simulink library "SignalPreprocessingLib"  (R2020b)
settings: Solver=VariableStepAuto  StartTime=0.0  StopTime=10.0  RelTol=1e-3
undefined symbols (not defined in the file or in its folder): fdesignblkfcn, fs, gcbh, param_ecg_gain_mv
(part 1 of 7)
settings Model: Creator=Rafael  LastModifiedBy=Rafael

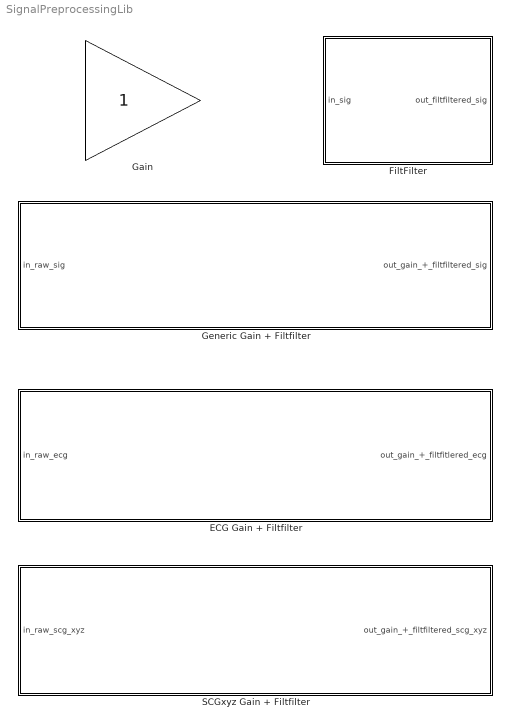
== system SignalPreprocessingLib ==
  ECG Gain + Filtfilter : Subsystem  mask{param_ecg_gain_mv=1000, param_ecg_fc_lo=2.05, param_ecg_fc_hi=36, param_ecg_trans_bw=2, param_plotflag=on}
      mask prompts: param_ecg_gain_mv "mV Conversion Gain"; param_ecg_fc_lo "Low Passband Frequency Corner (Hz)"; param_ecg_fc_hi "High Passband Frequency Corner (Hz)"; param_ecg_trans_bw "Transition Bandwidth (Hz)"; param_plotflag "Plot Flag"
      mask init:
      | assignin('base','param_ecg_gain_mv',param_ecg_gain_mv)
      | assignin('base','param_ecg_fc_lo',param_ecg_fc_lo)
      | assignin('base','param_ecg_fc_hi',param_ecg_fc_hi)
      | assignin('base','param_ecg_trans_bw',param_ecg_trans_bw)
      mask DialogControl DescGroupVar Prompt: ECG Preprocessing
      mask DialogControl DescTextVar Prompt: Preprocessing stage of the ECG. This involves conversion from V to mV and a filtfilt operation (i.e. a zero-phase FIR filtering) specified by the passband cornerns and transition bandwidth.
      mask Display: image('$imagefile'); % Use "Edit Image" on toolstrip to change.
  FiltFilter : Subsystem  mask{param_gain=1000, param_fc_lo=2.05, param_fc_hi=36, param_trans_bw=2, param_plotflag=on}
      mask prompts: param_gain "Gain"; param_fc_lo "Low Passband Frequency Corner (Hz)"; param_fc_hi "High Passband Frequency Corner (Hz)"; param_trans_bw "Transition Bandwidth (Hz)"; param_plotflag "Plot Flag"
      mask init:
      | assignin('base','param_gain_mv',param_gain)
      | assignin('base','param_fc_lo',param_fc_lo)
      | assignin('base','param_fc_hi',param_fc_hi)
      | assignin('base','param_trans_bw',param_trans_bw)
      mask DialogControl DescGroupVar Prompt: Signal  Preprocessing
      mask DialogControl DescTextVar Prompt: Preprocessing of a generica signal 'sig'. This involves a gain stage followed by a filtfilt operation (i.e. a zero-phase FIR filtering) specified by the passband cornerns and transition bandwidth.
      mask Display: image('Filtfilt.png'); % Use "Edit Image" on toolstrip to change.
  Gain : Gain
  Generic Gain + Filtfilter : Subsystem  mask{param_gain=1000, param_fc_lo=2.05, param_fc_hi=36, param_trans_bw=2, param_plotflag=on}
      mask prompts: param_gain "Gain"; param_fc_lo "Low Passband Frequency Corner (Hz)"; param_fc_hi "High Passband Frequency Corner (Hz)"; param_trans_bw "Transition Bandwidth (Hz)"; param_plotflag "Plot Flag"
      mask init:
      | assignin('base','param_gain_mv',param_gain)
      | assignin('base','param_fc_lo',param_fc_lo)
      | assignin('base','param_fc_hi',param_fc_hi)
      | assignin('base','param_trans_bw',param_trans_bw)
      mask DialogControl DescGroupVar Prompt: Signal  Preprocessing
      mask DialogControl DescTextVar Prompt: Preprocessing of a generica signal 'sig'. This involves a gain stage followed by a filtfilt operation (i.e. a zero-phase FIR filtering) specified by the passband cornerns and transition bandwidth.
      mask Display: image('$imagefile'); % Use "Edit Image" on toolstrip to change.
  SCGxyz Gain + Filtfilter : Subsystem  mask{param_scg_gain_mg=3333, param_scg_fc_lo=5, param_scg_fc_hi=120, param_scg_trans_bw=2.5, param_plotflag=on}
      mask prompts: param_scg_gain_mg "V to mg Conversion Gain"; param_scg_fc_lo "Low Passband Frequency Corner (Hz)"; param_scg_fc_hi "High Passband Frequency Corner (Hz)"; param_scg_trans_bw "Transition bandwidth"; param_plotflag "Plot Flag"
      mask init:
      | assignin('base','param_scg_gain_mg',param_scg_gain_mg)
      | assignin('base','param_scg_fc_lo',param_scg_fc_lo)
      | assignin('base','param_scg_fc_hi',param_scg_fc_hi)
      | assignin('base','param_scg_trans_bw',param_scg_trans_bw)
      mask DialogControl DescGroupVar Prompt: SCG Preprocessing
      mask DialogControl DescTextVar Prompt: The SCG (x, y, and z) preprocessing block. This involves a V to mg conversion (determined by the transducer sensitivity) and a filtfilt operation. This filtfilt operation consists of a zero-phase FIR front-back filtering that is identical for each of the three cartesian acceleration components and is specified by the passband frequency corners and the transition bandwidth.
      mask Display: image('SCGPreprocessingSymbol.png'); % Use "Edit Image" on toolstrip to change.

== system SignalPreprocessingLib/ECG Gain + Filtfilter ==
  in_raw_ecg : Inport
  Enabled ECG Preprocessing Subsystem : Subsystem  TreatAsAtomicUnit=on
  out_gain_+_filtfitlered_ecg : Outport  VectorParamsAs1DForOutWhenUnconnected=off
  wires:
  Enabled ECG Preprocessing Subsystem/1(out_gain_filtfiltered_ecg) -> out_gain_+_filtfitlered_ecg/1
  in_raw_ecg/1 -> Enabled ECG Preprocessing Subsystem/Enable

== system SignalPreprocessingLib/FiltFilter ==
  in_sig : Inport
  Enabled Filtfiltering Subsystem : Subsystem  TreatAsAtomicUnit=on
  out_filtfiltered_sig : Outport  VectorParamsAs1DForOutWhenUnconnected=off
  wires:
  Enabled Filtfiltering Subsystem/1(out_sig) -> out_filtfiltered_sig/1
  in_sig/1 -> Enabled Filtfiltering Subsystem/Enable

== system SignalPreprocessingLib/Generic Gain + Filtfilter ==
  in_raw_sig : Inport
  Enabled Sig Preprocessing Subsystem : Subsystem  TreatAsAtomicUnit=on
  out_gain_+_filtfiltered_sig : Outport  VectorParamsAs1DForOutWhenUnconnected=off
  wires:
  in_raw_sig/1 -> Enabled Sig Preprocessing Subsystem/Enable
  Enabled Sig Preprocessing Subsystem/1(out_gain_filtfiltered_sig) -> out_gain_+_filtfiltered_sig/1

== system SignalPreprocessingLib/SCGxyz Gain + Filtfilter ==
  in_raw_scg_xyz : Inport
  Enabled SCG Preprocessing Subsystem : Subsystem  TreatAsAtomicUnit=on
  out_gain_+_filtfiltered_scg_xyz : Outport  VectorParamsAs1DForOutWhenUnconnected=off
  wires:
  Enabled SCG Preprocessing Subsystem/1(out_gain_filtfilt_scg_xyz) -> out_gain_+_filtfiltered_scg_xyz/1
  in_raw_scg_xyz/1 -> Enabled SCG Preprocessing Subsystem/Enable

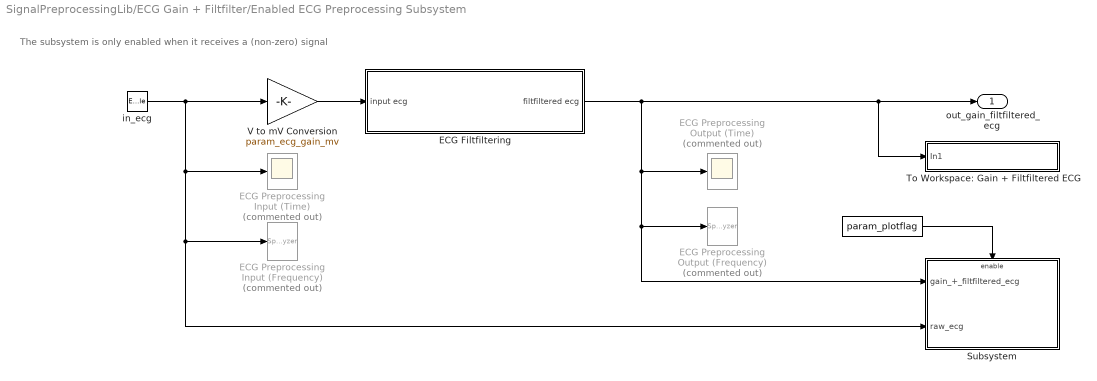
== system SignalPreprocessingLib/ECG Gain + Filtfilter/Enabled ECG Preprocessing Subsystem ==
  note: The subsystem is only enabled when it receives a (non-zero) signal
  in_ecg : EnablePort  ShowOutputPort=on
  " " : Constant  Value=param_plotflag
  ECG Filtfiltering : Subsystem
  ECG Preprocessing Input (Frequency) : SpectrumAnalyzer  Commented=on
  ECG Preprocessing Input (Time) : Scope  Commented=on
  ECG Preprocessing Output (Frequency) : SpectrumAnalyzer  Commented=on
  ECG Preprocessing Output (Time) : Scope  Commented=on
  Subsystem : Subsystem
  To Workspace: Gain + Filtfiltered ECG : Subsystem
      mask Display: disp('out_gain_+_filfiltered_ecg')
  V to mV Conversion : Gain  Gain=param_ecg_gain_mv
  out_gain_filtfiltered_ecg : Outport  VectorParamsAs1DForOutWhenUnconnected=off
  wires:
  V to mV Conversion/1 -> ECG Filtfiltering/1(input ecg)
  in_ecg/1 -> V to mV Conversion/1, ECG Preprocessing Input (Time)/1, Subsystem/2(raw_ecg), ECG Preprocessing Input (Frequency)/1
  ECG Filtfiltering/1(filtfiltered ecg) -> out_gain_filtfiltered_ecg/1, To Workspace: Gain + Filtfiltered ECG/1(In1), ECG Preprocessing Output (Time)/1, ECG Preprocessing Output (Frequency)/1, Subsystem/1(gain_+_filtfiltered_ecg)
  " "/1 -> Subsystem/Enable

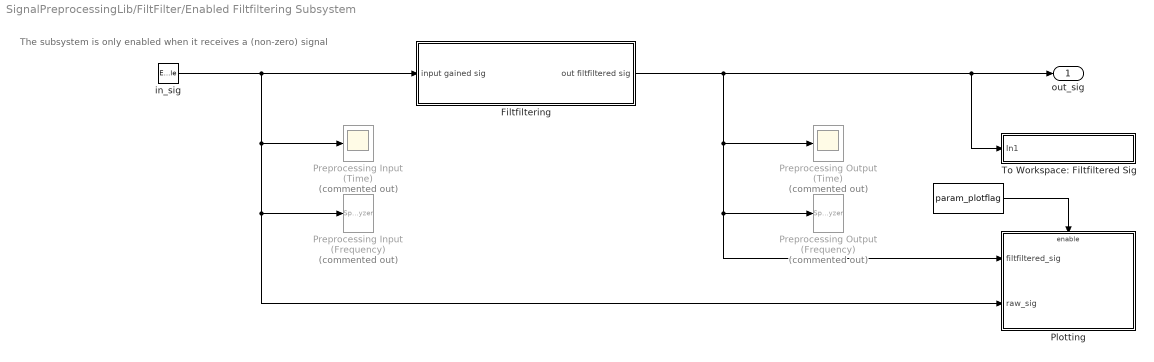
== system SignalPreprocessingLib/FiltFilter/Enabled Filtfiltering Subsystem ==
  note: The subsystem is only enabled when it receives a (non-zero) signal
  in_sig : EnablePort  ShowOutputPort=on
  " " : Constant  Value=param_plotflag
  Filtfiltering : Subsystem
  Plotting : Subsystem
  Preprocessing Input (Frequency) : SpectrumAnalyzer  Commented=on
  Preprocessing Input (Time) : Scope  Commented=on
  Preprocessing Output (Frequency) : SpectrumAnalyzer  Commented=on
  Preprocessing Output (Time) : Scope  Commented=on
  To Workspace: Filtfiltered Sig : Subsystem
      mask Display: disp('out_sig_filtfiltered')
  out_sig : Outport  VectorParamsAs1DForOutWhenUnconnected=off
  wires:
  in_sig/1 -> Filtfiltering/1(input gained sig), Preprocessing Input (Time)/1, Plotting/2(raw_sig), Preprocessing Input (Frequency)/1
  Filtfiltering/1(out filtfiltered sig) -> To Workspace: Filtfiltered Sig/1(In1), out_sig/1, Preprocessing Output (Time)/1, Plotting/1(filtfiltered_sig), Preprocessing Output (Frequency)/1
  " "/1 -> Plotting/Enable

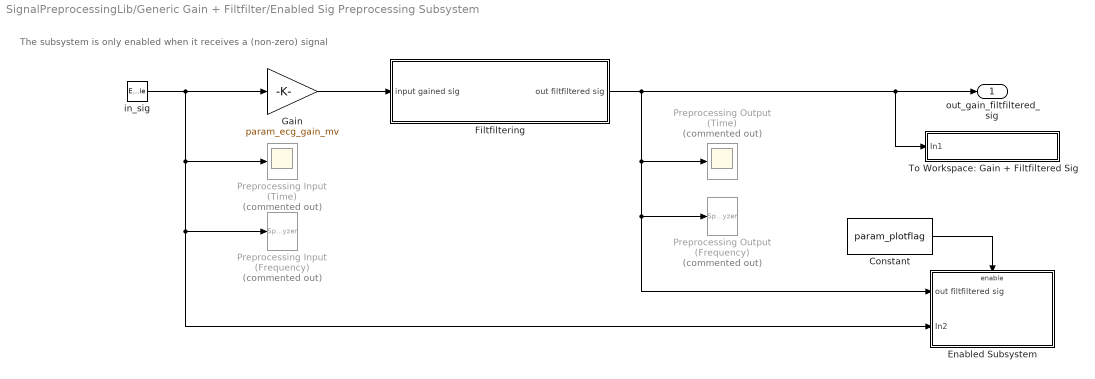
== system SignalPreprocessingLib/Generic Gain + Filtfilter/Enabled Sig Preprocessing Subsystem ==
  note: The subsystem is only enabled when it receives a (non-zero) signal
  in_sig : EnablePort  ShowOutputPort=on
  Constant : Constant  Value=param_plotflag
  Enabled Subsystem : Subsystem  TreatAsAtomicUnit=on
  Filtfiltering : Subsystem
  Gain : Gain  Gain=param_ecg_gain_mv
  Preprocessing Input (Frequency) : SpectrumAnalyzer  Commented=on
  Preprocessing Input (Time) : Scope  Commented=on
  Preprocessing Output (Frequency) : SpectrumAnalyzer  Commented=on
  Preprocessing Output (Time) : Scope  Commented=on
  To Workspace: Gain + Filtfiltered Sig : Subsystem
      mask Display: disp('out_gain_+_filfiltered_sig')
  out_gain_filtfiltered_sig : Outport  VectorParamsAs1DForOutWhenUnconnected=off
  wires:
  Filtfiltering/1(out filtfiltered sig) -> Enabled Subsystem/1(out filtfiltered sig), Preprocessing Output (Frequency)/1, Preprocessing Output (Time)/1, out_gain_filtfiltered_sig/1, To Workspace: Gain + Filtfiltered Sig/1(In1)
  in_sig/1 -> Enabled Subsystem/2(In2), Preprocessing Input (Frequency)/1, Preprocessing Input (Time)/1, Gain/1
  Gain/1 -> Filtfiltering/1(input gained sig)
  Constant/1 -> Enabled Subsystem/Enable

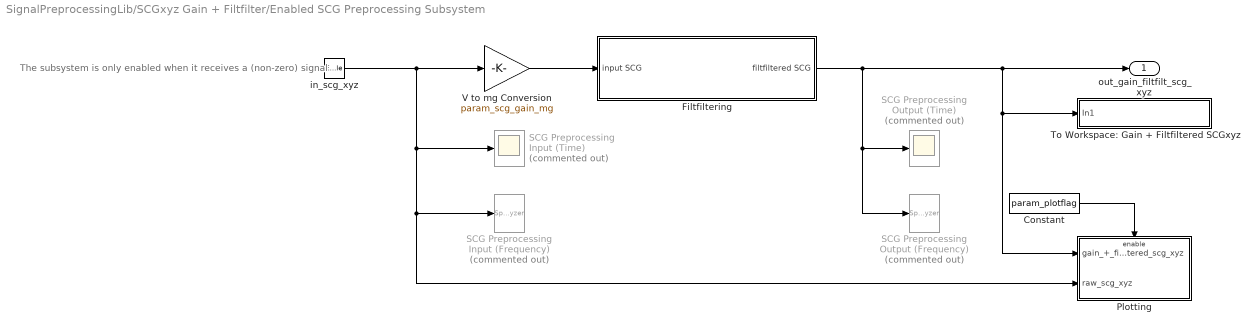
== system SignalPreprocessingLib/SCGxyz Gain + Filtfilter/Enabled SCG Preprocessing Subsystem ==
  note: The subsystem is only enabled when it receives a (non-zero) signal
  in_scg_xyz : EnablePort  ShowOutputPort=on
  Constant : Constant  Value=param_plotflag
  Filtfiltering : Subsystem
  Plotting : Subsystem
  SCG Preprocessing Input (Frequency) : SpectrumAnalyzer  Commented=on
  SCG Preprocessing Input (Time) : Scope  Commented=on
  SCG Preprocessing Output (Frequency) : SpectrumAnalyzer  Commented=on
  SCG Preprocessing Output (Time) : Scope  Commented=on
  To Workspace: Gain + Filtfiltered SCGxyz : Subsystem
      mask Display: disp('out_gain_+_filfiltered_scgxyz')
  V to mg Conversion : Gain  Gain=param_scg_gain_mg
  out_gain_filtfilt_scg_xyz : Outport  VectorParamsAs1DForOutWhenUnconnected=off
  wires:
  V to mg Conversion/1 -> Filtfiltering/1(" input SCG")
  Filtfiltering/1(filtfiltered SCG) -> out_gain_filtfilt_scg_xyz/1, Plotting/1(gain_+_filtfiltered_scg_xyz), To Workspace: Gain + Filtfiltered SCGxyz/1(In1), SCG Preprocessing Output (Frequency)/1, SCG Preprocessing Output (Time)/1
  in_scg_xyz/1 -> V to mg Conversion/1, Plotting/2(raw_scg_xyz), SCG Preprocessing Input (Frequency)/1, SCG Preprocessing Input (Time)/1
  Constant/1 -> Plotting/Enable

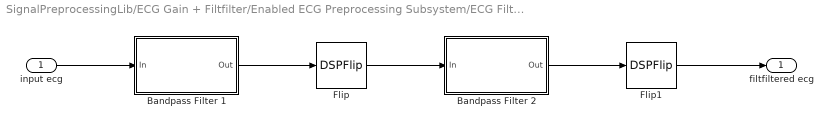
== system SignalPreprocessingLib/ECG Gain + Filtfilter/Enabled ECG Preprocessing Subsystem/ECG Filtfiltering ==
  input ecg : Inport
  Bandpass Filter 1 : Subsystem  DialogController=fdesignblkfcn  InitFcn=fdesignblkfcn(gcbh, {'InitFcn'});  mask(Bandpass Filter){}
      mask help: Design a bandpass filter
      settings: CopyFcn=fdesignblkfcn(gcbh, {'CopyFcn'});
      mask Help: helpview(mapfilelocation('dsp'), 'dspbandpassfilter');
      mask Display: disp('Bandpass');
  Bandpass Filter 2 : Subsystem  DialogController=fdesignblkfcn  InitFcn=fdesignblkfcn(gcbh, {'InitFcn'});  mask(Bandpass Filter){}
      mask help: Design a bandpass filter
      settings: CopyFcn=fdesignblkfcn(gcbh, {'CopyFcn'});
      mask Help: helpview(mapfilelocation('dsp'), 'dspbandpassfilter');
      mask Display: disp('Bandpass');
  Flip : DSPFlip
  Flip1 : DSPFlip
  filtfiltered ecg : Outport  VectorParamsAs1DForOutWhenUnconnected=off
  wires:
  Flip/1 -> Bandpass Filter 2/1(In)
  input ecg/1 -> Bandpass Filter 1/1(In)
  Flip1/1 -> filtfiltered ecg/1
  Bandpass Filter 1/1(Out) -> Flip/1
  Bandpass Filter 2/1(Out) -> Flip1/1

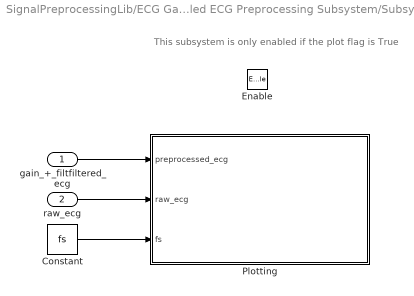
== system SignalPreprocessingLib/ECG Gain + Filtfilter/Enabled ECG Preprocessing Subsystem/Subsystem ==
  note: This subsystem is only enabled if the plot flag is True
  gain_+_filtfiltered_ecg : Inport
  raw_ecg : Inport  Port=2
  Enable : EnablePort
  Constant : Constant  Value=fs
  Plotting : MATLAB Function  TreatAsAtomicUnit=on
  wires:
  Constant/1 -> Plotting/3(fs)
  gain_+_filtfiltered_ecg/1 -> Plotting/1(preprocessed_ecg)
  raw_ecg/1 -> Plotting/2(raw_ecg)

== system SignalPreprocessingLib/ECG Gain + Filtfilter/Enabled ECG Preprocessing Subsystem/To Workspace: Gain + Filtfiltered ECG ==
  In1 : Inport
  Enabled To Workspace Subsystem : Subsystem  TreatAsAtomicUnit=on
  wires:
  In1/1 -> Enabled To Workspace Subsystem/Enable, Enabled To Workspace Subsystem/1(In1)

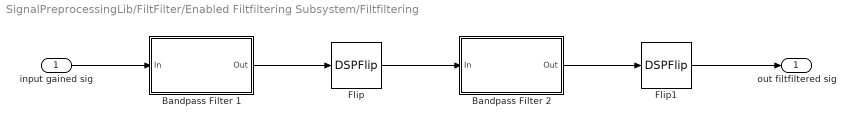
== system SignalPreprocessingLib/FiltFilter/Enabled Filtfiltering Subsystem/Filtfiltering ==
  input gained sig : Inport
  Bandpass Filter 1 : Subsystem  DialogController=fdesignblkfcn  InitFcn=fdesignblkfcn(gcbh, {'InitFcn'});  mask(Bandpass Filter){}
      mask help: Design a bandpass filter
      settings: CopyFcn=fdesignblkfcn(gcbh, {'CopyFcn'});
      mask Help: helpview(mapfilelocation('dsp'), 'dspbandpassfilter');
      mask Display: disp('Bandpass');
  Bandpass Filter 2 : Subsystem  DialogController=fdesignblkfcn  InitFcn=fdesignblkfcn(gcbh, {'InitFcn'});  mask(Bandpass Filter){}
      mask help: Design a bandpass filter
      settings: CopyFcn=fdesignblkfcn(gcbh, {'CopyFcn'});
      mask Help: helpview(mapfilelocation('dsp'), 'dspbandpassfilter');
      mask Display: disp('Bandpass');
  Flip : DSPFlip
  Flip1 : DSPFlip
  out filtfiltered sig : Outport  VectorParamsAs1DForOutWhenUnconnected=off
  wires:
  Flip/1 -> Bandpass Filter 2/1(In)
  input gained sig/1 -> Bandpass Filter 1/1(In)
  Flip1/1 -> out filtfiltered sig/1
  Bandpass Filter 1/1(Out) -> Flip/1
  Bandpass Filter 2/1(Out) -> Flip1/1

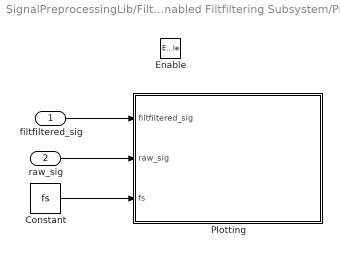
== system SignalPreprocessingLib/FiltFilter/Enabled Filtfiltering Subsystem/Plotting ==
  filtfiltered_sig : Inport
  raw_sig : Inport  Port=2
  Enable : EnablePort
  Constant : Constant  Value=fs
  Plotting : MATLAB Function  TreatAsAtomicUnit=on
  wires:
  Constant/1 -> Plotting/3(fs)
  filtfiltered_sig/1 -> Plotting/1(filtfiltered_sig)
  raw_sig/1 -> Plotting/2(raw_sig)

== system SignalPreprocessingLib/FiltFilter/Enabled Filtfiltering Subsystem/To Workspace: Filtfiltered Sig ==
  In1 : Inport
  Enabled To Workspace Subsystem : Subsystem  TreatAsAtomicUnit=on
  wires:
  In1/1 -> Enabled To Workspace Subsystem/Enable, Enabled To Workspace Subsystem/1(In1)

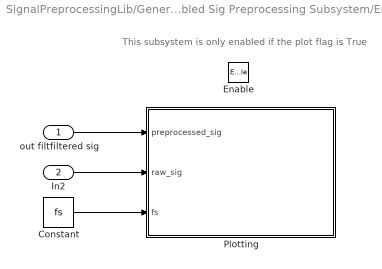
== system SignalPreprocessingLib/Generic Gain + Filtfilter/Enabled Sig Preprocessing Subsystem/Enabled Subsystem ==
  note: This subsystem is only enabled if the plot flag is True
  out filtfiltered sig : Inport
  In2 : Inport  Port=2
  Enable : EnablePort
  Constant : Constant  Value=fs
  Plotting : MATLAB Function  TreatAsAtomicUnit=on
  wires:
  Constant/1 -> Plotting/3(fs)
  out filtfiltered sig/1 -> Plotting/1(preprocessed_sig)
  In2/1 -> Plotting/2(raw_sig)

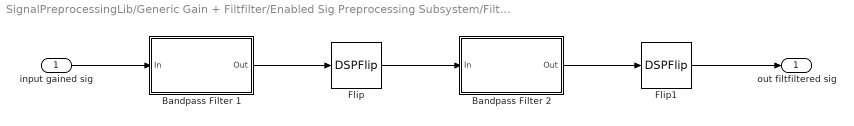
== system SignalPreprocessingLib/Generic Gain + Filtfilter/Enabled Sig Preprocessing Subsystem/Filtfiltering ==
  input gained sig : Inport
  Bandpass Filter 1 : Subsystem  DialogController=fdesignblkfcn  InitFcn=fdesignblkfcn(gcbh, {'InitFcn'});  mask(Bandpass Filter){}
      mask help: Design a bandpass filter
      settings: CopyFcn=fdesignblkfcn(gcbh, {'CopyFcn'});
      mask Help: helpview(mapfilelocation('dsp'), 'dspbandpassfilter');
      mask Display: disp('Bandpass');
  Bandpass Filter 2 : Subsystem  DialogController=fdesignblkfcn  InitFcn=fdesignblkfcn(gcbh, {'InitFcn'});  mask(Bandpass Filter){}
      mask help: Design a bandpass filter
      settings: CopyFcn=fdesignblkfcn(gcbh, {'CopyFcn'});
      mask Help: helpview(mapfilelocation('dsp'), 'dspbandpassfilter');
      mask Display: disp('Bandpass');
  Flip : DSPFlip
  Flip1 : DSPFlip
  out filtfiltered sig : Outport  VectorParamsAs1DForOutWhenUnconnected=off
  wires:
  Bandpass Filter 2/1(Out) -> Flip1/1
  Bandpass Filter 1/1(Out) -> Flip/1
  Flip1/1 -> out filtfiltered sig/1
  input gained sig/1 -> Bandpass Filter 1/1(In)
  Flip/1 -> Bandpass Filter 2/1(In)

== system SignalPreprocessingLib/Generic Gain + Filtfilter/Enabled Sig Preprocessing Subsystem/To Workspace: Gain + Filtfiltered Sig ==
  In1 : Inport
  Enabled To Workspace Subsystem : Subsystem  TreatAsAtomicUnit=on
  wires:
  In1/1 -> Enabled To Workspace Subsystem/1(In1), Enabled To Workspace Subsystem/Enable

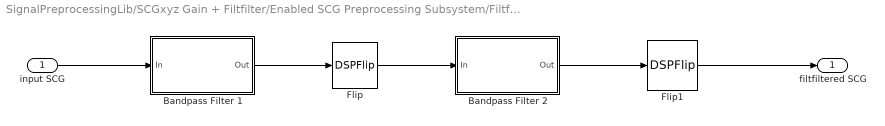
== system SignalPreprocessingLib/SCGxyz Gain + Filtfilter/Enabled SCG Preprocessing Subsystem/Filtfiltering ==
  " input SCG" : Inport
  Bandpass Filter 1 : Subsystem  DialogController=fdesignblkfcn  InitFcn=fdesignblkfcn(gcbh, {'InitFcn'});  mask(Bandpass Filter){}
      mask help: Design a bandpass filter
      settings: CopyFcn=fdesignblkfcn(gcbh, {'CopyFcn'});
      mask Help: helpview(mapfilelocation('dsp'), 'dspbandpassfilter');
      mask Display: disp('Bandpass');
  Bandpass Filter 2 : Subsystem  DialogController=fdesignblkfcn  InitFcn=fdesignblkfcn(gcbh, {'InitFcn'});  mask(Bandpass Filter){}
      mask help: Design a bandpass filter
      settings: CopyFcn=fdesignblkfcn(gcbh, {'CopyFcn'});
      mask Help: helpview(mapfilelocation('dsp'), 'dspbandpassfilter');
      mask Display: disp('Bandpass');
  Flip : DSPFlip
  Flip1 : DSPFlip
  filtfiltered SCG : Outport  VectorParamsAs1DForOutWhenUnconnected=off
  wires:
  Bandpass Filter 2/1(Out) -> Flip1/1
  Bandpass Filter 1/1(Out) -> Flip/1
  Flip1/1 -> filtfiltered SCG/1
  " input SCG"/1 -> Bandpass Filter 1/1(In)
  Flip/1 -> Bandpass Filter 2/1(In)

== system SignalPreprocessingLib/SCGxyz Gain + Filtfilter/Enabled SCG Preprocessing Subsystem/Plotting ==
  note: This subsystem is only enabled when the plot falg is True
  gain_+_filtfiltered_scg_xyz : Inport
  raw_scg_xyz : Inport  Port=2
  Enable : EnablePort
  Constant : Constant  Value=fs
  Plotting : MATLAB Function  TreatAsAtomicUnit=on
  wires:
  Constant/1 -> Plotting/3(fs)
  raw_scg_xyz/1 -> Plotting/2(raw_scg_xyz)
  gain_+_filtfiltered_scg_xyz/1 -> Plotting/1(gain_filtfiltered_scg_xyz)

== system SignalPreprocessingLib/SCGxyz Gain + Filtfilter/Enabled SCG Preprocessing Subsystem/To Workspace: Gain + Filtfiltered SCGxyz ==
  In1 : Inport
  To Workspace Enabled Subsystem : Subsystem  TreatAsAtomicUnit=on
  wires:
  In1/1 -> To Workspace Enabled Subsystem/Enable, To Workspace Enabled Subsystem/1(In1)

== system SignalPreprocessingLib/ECG Gain + Filtfilter/Enabled ECG Preprocessing Subsystem/ECG Filtfiltering/Bandpass Filter 1 ==
  In : Inport
  Generated Filter Block : DiscreteFir  Tag=BlockMethodSubSystem  Coefficients=[-0.0114243088354877773 0.00587624110456374388 0.00413946068324517157 0.00264334557424035672 0.00138774422276622192 0.00039597756815762733 -0.000357391963790950132 -0.000870027328167087902 -0.00118474210009046274 -0.0013114772414377189 -0.00130211118137258525 -0.00117028348293094116 -0.000969555288066135598 -0.000709991739662891794 -0.000441672338585462343 -0.000165596169411169614 7.38618239838010476e-05 0.000289182992126718261 0.00043918297873611449 0.000554539538172022298 0.000596791094711021305 0.000591852861038305242 0.000558642096174625374 0.000449318410474004379 0.000334719809825502479 0.00020575650819831294 5.39363215079843861e-05 -0.000101322531501510382 -0.000240833690149395291 -0.000354646039305753225 -0.000451018706232981029 -0.000523127741752206499 -0.000570171746042747937 -0.000579976289078059509 -0.000560050610609794802 -0.000510203484091005868 -0.000444253999700439106 -0.000361620699264023418 -0.000270418439597897714 -0.000171285996548194847 -6.96491449474114649e-05 2.51074882581126674e-05 0.000107701466472475207 0.000177443554931332875 0.000215288445749358542 0.000245848468855064048 0.000245696970898627229 0.000229649686627229205 0.00019096241212286473 0.000142984412950488554 7.04459950623022302e-05 -8.24128026295257998e-06 -9.80593727097200246e-05 -0.000181512369773678683 -0.000268731962362029828 -0.000342263684306691809 -0.000409113387221587271 -0.000453067377901137172 -0.000486836085121275519 -0.000497275928952340546 -0.00049828288783324709 -0.000472232231767717378 -0.00043821960462679492 -0.000378588991066479766 -0.000316844305738618603 -0.000241178452312015845 -0.000166037327502541535 -8.72939132895780845e-05 -1.92312446675550752e-05 4.72061762121969014e-05 9.32922079647201252e-05 0.000128677828260322091 0.000142225646220916352 0.000145392718308013161 0.000124316294889322346 9.22525950362868691e-05 3.91139366419743922e-05 -2.09540055264127723e-05 -9.84817072707550728e-05 -0.000176447200533612 -0.000261969930569216219 -0.000338398170707415388 -0.000413673787246831778 -0.000474956484152477126 -0.000526126847064748229 -0.000557031780194342657 -0.000573463759814568652 -0.000565518328802135789 -0.000545968260267525388 -0.000503292825521842527 -0.000450686144492560767 -0.00038193732270500047 -0.000310533512604118864 -0.000229221000311531989 -0.000153634622944792687 -7.7008709436998668e-05 -1.29951882972875049e-05 4.41972427699440645e-05 7.97744827227258452e-05 0.000101355022460052069 9.88614688825825011e-05 8.13696224336354218e-05 3.98982051577762009e-05 -1.42484593806998378e-05 -8.82654671942838254e-05 -0.000167074457359766074 -0.00025963077237387 -0.000347989994374806391 -0.000439444994547399936 -0.00051811479354047299 -0.000590082617058047473 -0.000641838802120880611 -0.000681503522967578934 -0.000694804478821137508 -0.00069209853970065606 -0.000663795693677639645 -0.000621757222242421206 -0.000557224399686986893 -0.000484587241980041772 -0.000396687438130890677 -0.000308737174406251494 -0.000214743893139471981 -0.00013218336614707546 -5.38482479860227792e-05 3.99111044497961476e-06 4.92154210607297082e-05 6.74354760492514721e-05 6.74472479585495194e-05 4.02217001782036176e-05 -4.06942016077313506e-06 -7.33562872444193381e-05 -0.000154074998390272069 -0.000252782754343081062 -0.000354062465090758047 -0.000462222943123069205 -0.000562271536985421011 -0.000658661832374597689 -0.000735808311790427799 -0.000799943578584080828 -0.000838241882526128551 -0.000857844739487072239 -0.000847533102258754556 -0.000817418121589637975 -0.000760200301916437102 -0.000687422833072246636 -0.000595027809558780832 -0.000496080524377292761 -0.000387710990138089018 -0.000284208196984854847 -0.000182518571703508756 -9.84384035011120345e-05 -2.73607674165961268e-05 1.77508990696524649e-05 4.21653277528823839e-05 3.53040248291924125e-05 5.59921773045889137e-06 -5.46825757556310132e-05 -0.000133739024050423885 -0.000236066993422962002 -0.000348549704079315764 -0.000473403235651745358 -0.000595572390038458938 -0.000716976323207035166 ...(+20655 chars)]  InputProcessing=Columns as channels (frame based)
  Out : Outport  VectorParamsAs1DForOutWhenUnconnected=off
  wires:
  In/1 -> Generated Filter Block/1
  Generated Filter Block/1 -> Out/1
